simulink subsystem "classification"  (R2025b)
settings: Solver=VariableStepAuto  StartTime=0.0  StopTime=10.0  RelTol=1e-3
libraries: dspstat3 x2, simulink x1
settings Model: Creator=sanborkl  LastModifiedBy=sanborkl

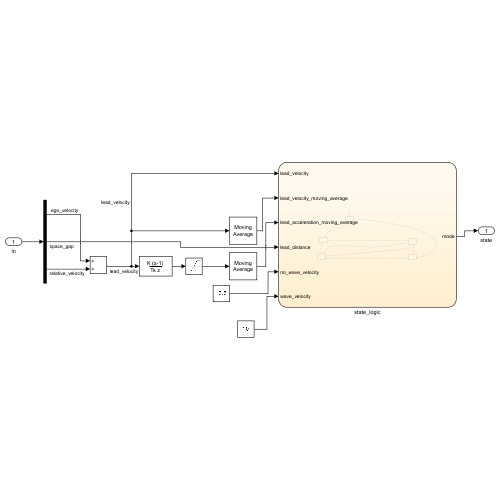
[thumbnail: Simulink's stored preview of the top-level diagram]
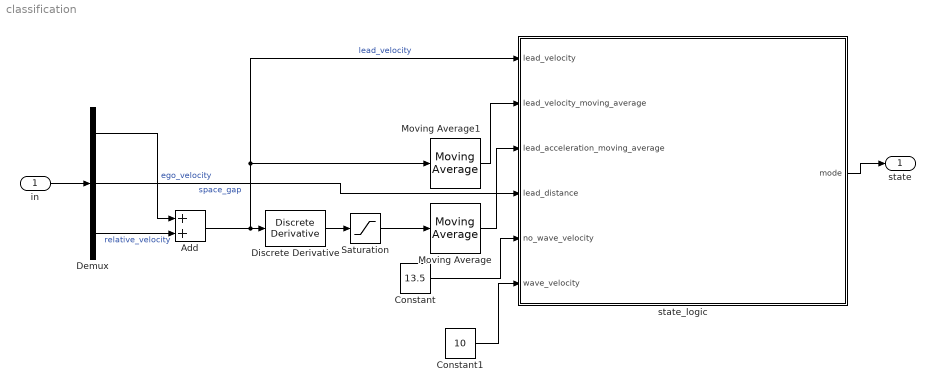
== system classification ==
  in : Inport
  Add : Sum
  Constant : Constant  Value=13.5
  Constant1 : Constant  Value=10
  Demux : Demux  Outputs=3
  Discrete Derivative : simulink/Discrete/Discrete Derivative  gainval=1.0  ICPrevScaledInput=0.0  OutMin=[]  OutMax=[3]  OutDataType=fixdt(1, 16)  OutScaling=2^-10  DoSatur=off
  Moving Average : dspstat3/Moving Average  Method=Sliding window  ForgettingFactorPort=off  SpecifyWindowLength=on  WindowLength=10  OverlapLength=10 - 1  AllowArbitraryInputLength=off  ForgettingFactor=0.9  SimulateUsing=Interpreted execution
  Moving Average1 : dspstat3/Moving Average  Method=Sliding window  ForgettingFactorPort=off  SpecifyWindowLength=on  WindowLength=10  OverlapLength=10 - 1  AllowArbitraryInputLength=off  ForgettingFactor=0.9  SimulateUsing=Interpreted execution
  Saturation : Saturate  UpperLimit=2.0  LowerLimit=-3.5
  state_logic : Stateflow chart  TreatAsAtomicUnit=on
  state : Outport
  wires:
  in/1 -> Demux/1
  Demux/3 -> Add/2  "relative_velocity"
  Demux/1 -> Add/1  "ego_velocity"
  Moving Average/1 -> state_logic/3(lead_acceleration_moving_average)
  state_logic/1(mode) -> state/1
  Moving Average1/1 -> state_logic/2(lead_velocity_moving_average)
  Add/1 -> Discrete Derivative/1, Moving Average1/1, state_logic/1(lead_velocity)  "lead_velocity"
  Discrete Derivative/1 -> Saturation/1
  Saturation/1 -> Moving Average/1
  Demux/2 -> state_logic/4(lead_distance)  "space_gap"
  Constant/1 -> state_logic/5(no_wave_velocity)
  Constant1/1 -> state_logic/6(wave_velocity)

== stateflow chart classification/state_logic ==
  note: 13.5 m/s ~ 30 mph
      | 10 m/s ~ 22 mph
  state intial
  state no_wave
    mode = 0;
  state into_wave
    mode = 1;
  state out_of_wave
    mode = 3;
  state in_wave
    mode = 2;
  (default) -> intial
  intial -> in_wave [order 2] : [lead_velocity <= no_wave_velocity & lead_distance <= 200]
  intial -> no_wave [order 1] : [lead_velocity > no_wave_velocity | lead_distance > 200]
  no_wave -> into_wave : [(lead_acceleration_moving_average < -0.5 & lead_velocity < no_wave_velocity & lead_distance < 200) | (lead_velocity < no_wave_velocity & lead_distance < 75)]
  out_of_wave -> no_wave [order 1] : [lead_velocity_moving_average > no_wave_velocity]
  into_wave -> out_of_wave [order 2] : [lead_acceleration_moving_average >= 0.25]
  out_of_wave -> into_wave [order 2] : [lead_acceleration_moving_average <= -0.25]
  into_wave -> in_wave [order 1] : [lead_velocity_moving_average <= wave_velocity]
  in_wave -> out_of_wave : [lead_acceleration_moving_average > 0.5 & lead_velocity > wave_velocity]
  data: mode output; lead_velocity input; lead_velocity_moving_average input; lead_acceleration_moving_average input; lead_distance input; no_wave_velocity input; wave_velocity input
